simulink model "mass3"  (R2022a)
settings: Solver=FixedStepAuto  StartTime=0.0  StopTime=20  FixedStep=2e-5  RelTol=1e-3
values from neighbouring files (symbols this model uses):
  J2 = 0.12    [EDriveLab1.m]
undefined symbols (not defined in the file or in its folder): J1, K12
settings Model: Creator=Family  LastModifiedBy=Family

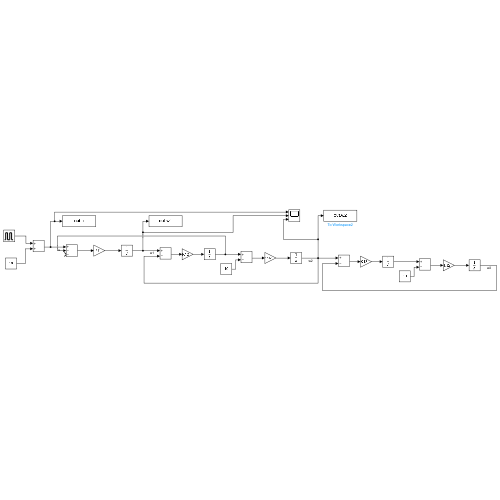
[thumbnail: Simulink's stored preview of the top-level diagram]
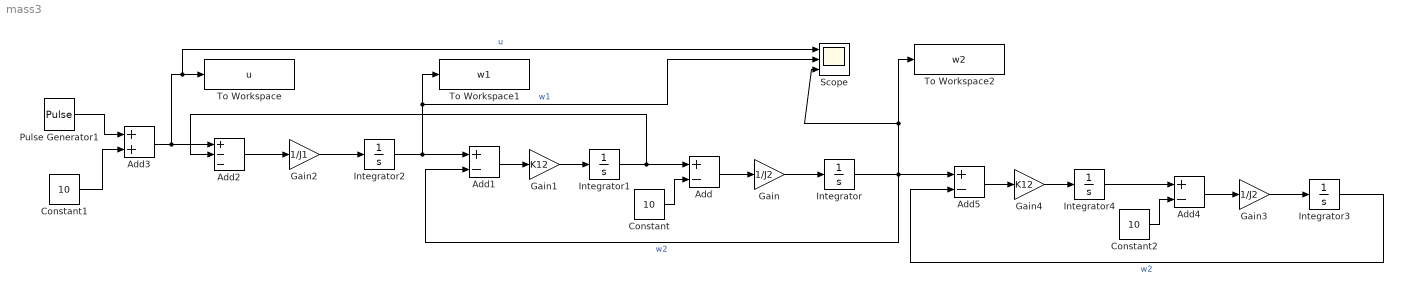
== system mass3 ==
  Add{,1,4..5} (4 alike) : Sum  Inputs=+-
  Add2 : Sum  Inputs=+--
  Add3 : Sum
  Constant : Constant  Value=10
  Constant1 : Constant  Value=10
  Constant2 : Constant  Value=10
  Gain : Gain  Gain=1/J2
  Gain1 : Gain  Gain=K12
  Gain2 : Gain  Gain=1/J1
  Gain3 : Gain  Gain=1/J2
  Gain4 : Gain  Gain=K12
  Integrator{,1..4} (5 alike) : Integrator
  Pulse Generator1 : DiscretePulseGenerator  PulseType=Time based  Amplitude=10  Period=5  PulseWidth=50
  Scope : Scope  NumInputPorts=3
  To Workspace : ToWorkspace  VariableName=u  SaveFormat=Timeseries  SampleTime=0.001
  To Workspace1 : ToWorkspace  VariableName=w1  SaveFormat=Timeseries  SampleTime=0.001
  To Workspace2 : ToWorkspace  VariableName=w2  SaveFormat=Timeseries  SampleTime=0.001
  wires:
  Gain/1 -> Integrator/1
  Add/1 -> Gain/1
  Integrator1/1 -> Add/1, Add2/2
  Gain1/1 -> Integrator1/1
  Add1/1 -> Gain1/1
  Integrator/1 -> Add5/1, Scope/3, To Workspace2/1, Add1/2  "w2"
  Integrator2/1 -> Add1/1, Scope/2, To Workspace1/1  "w1"
  Gain2/1 -> Integrator2/1
  Add2/1 -> Gain2/1
  Constant/1 -> Add/2
  Add3/1 -> Add2/1, Scope/1, To Workspace/1  "u"
  Pulse Generator1/1 -> Add3/1
  Constant1/1 -> Add3/2
  Integrator4/1 -> Add4/1
  Add4/1 -> Gain3/1
  Constant2/1 -> Add4/2
  Gain4/1 -> Integrator4/1
  Gain3/1 -> Integrator3/1
  Add5/1 -> Gain4/1
  Integrator3/1 -> Add5/2  "w2"
